simulink model "Altitude_control"  (R2016a)
settings: Solver=ode45  StartTime=0.0  StopTime=300.0  RelTol=1e-3
libraries: simulink_need_slupdate x1
settings Model: Creator=Jamie  LastModifiedBy=Jamie

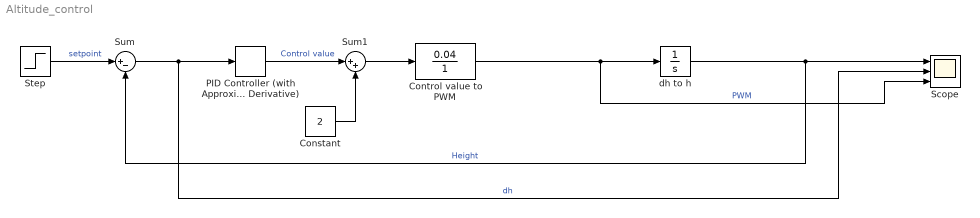
== system Altitude_control ==
  Constant : Constant  Value=2
  Control value to PWM : TransferFcn  Numerator=[0.04]  Denominator=[1]
  PID Controller (with Approximate Derivative) : simulink_need_slupdate/PID Controller (with Approximate Derivative)  P=1  I=0  D=0  N=100
  Scope : Scope  NumInputPorts=3
  Step : Step  After=50  SampleTime=0
  Sum : Sum  Inputs=|+-
  Sum1 : Sum  Inputs=|++
  dh to h : Integrator  InitialCondition=100
  wires:
  Step/1 -> Sum/1  "setpoint"
  Sum/1 -> PID Controller (with Approximate Derivative)/1, Scope/2  "dh"
  PID Controller (with Approximate Derivative)/1 -> Sum1/1  "Control value"
  dh to h/1 -> Sum/2, Scope/1  "Height"
  Constant/1 -> Sum1/2
  Sum1/1 -> Control value to PWM/1
  Control value to PWM/1 -> Scope/3, dh to h/1  "PWM"
